simulink library "xpcnilib"  (Simulink 6.0)
settings: Solver=ode45  SolverMode=SingleTasking  StartTime=0.0  StopTime=10.0  RelTol=1e-3
undefined symbols (not defined in the file or in its folder): madnipcie, mctrnipcie, mctrnipciecap, mdacbisa, mdanipci670x, mdanipci671x, mdanipcie, mdionipci6527, mdionipcie, mencnipci660x, misa8255, mnigpib, mnipci660x, mpci8255
libraries: xpcmeasurementcomputinglib x6
(part 1 of 3)
settings Model: Creator=adowd  LastModifiedBy=gweast
settings DataIOCC: SignalLoggingName=logsOut
settings OptimizationCC: BooleanDataType=off
settings DebuggingCC: CheckExecutionContextPreStartOutputMsg=on  CheckExecutionContextRuntimeOutputMsg=on  SolverPrmCheckMsg=none
settings HardwareCC: TargetUnknown=on
settings SFSimCC: SFSimApplyToAllLibs=on  SFSimBuildMode=Incremental

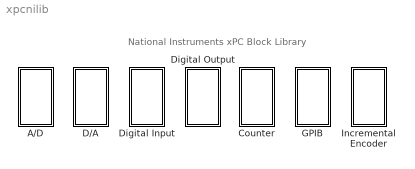
== system xpcnilib ==
  note: National Instruments xPC Block Library
  A/D : Subsystem  PropExecContextAcrossSSBoundary=on
  Counter : Subsystem  PropExecContextAcrossSSBoundary=on
  D/A : Subsystem  PropExecContextAcrossSSBoundary=on
  Digital Input : Subsystem  PropExecContextAcrossSSBoundary=on
  Digital Output : Subsystem  PropExecContextAcrossSSBoundary=on
  GPIB : Subsystem  PropExecContextAcrossSSBoundary=on
  Incremental Encoder : Subsystem  PropExecContextAcrossSSBoundary=on

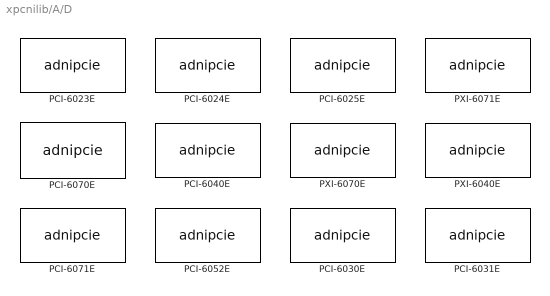
== system xpcnilib/A/D ==
  "PCI-6023E " : S-Function  InitFcn=madnipcie(1);  FunctionName=adnipcie  Parameters="channel, range, coupling, sampletime, slot,  boardType"  mask(adnipcie){channel=[1], range=[-10], coupling=[0], sampletime=0.001, slot=-1}
      mask prompts: channel "Channel vector:"; range "Range vector:"; coupling "Input coupling vector:"; sampletime "Sample time:"; slot "PCI slot (-1: autosearch):"
      mask help:
      | PCI-6023E
      | National Instruments
      | Analog Input
      mask init:
      | boardType=1;
      | madnipcie(2,channel, range, coupling, slot, boardType);
      mask Help: helpview(fullfile(docroot, 'mapfiles', 'xpc.map'), 'NationalInstruments_PCI-6023E_AD')
      mask Display: disp('PCI-6023E\nNational Instr.\nAnalog Input');port_label('output',1,'1');
  "PCI-6024E " : S-Function  InitFcn=madnipcie(1);  FunctionName=adnipcie  Parameters="channel, range, coupling, sampletime, slot,  boardType"  mask(adnipcie){channel=[1], range=[-10], coupling=[0], sampletime=0.001, slot=-1}
      mask prompts: channel "Channel vector:"; range "Range vector:"; coupling "Input coupling vector:"; sampletime "Sample time:"; slot "PCI slot (-1: autosearch):"
      mask help:
      | PCI-6024E
      | National Instruments
      | Analog Input
      mask init:
      | boardType=2;
      | madnipcie(2,channel, range, coupling, slot, boardType);
      mask Help: helpview(fullfile(docroot, 'mapfiles', 'xpc.map'), 'NationalInstruments_PCI-6024E_AD')
      mask Display: disp('PCI-6024E\nNational Instr.\nAnalog Input');port_label('output',1,'1');
  "PCI-6025E " : S-Function  InitFcn=madnipcie(1);  FunctionName=adnipcie  Parameters="channel, range, coupling, sampletime, slot,  boardType"  mask(adnipcie){channel=[1], range=[-10], coupling=[0], sampletime=0.001, slot=-1}
      mask prompts: channel "Channel vector:"; range "Range vector:"; coupling "Input coupling vector:"; sampletime "Sample time:"; slot "PCI slot (-1: autosearch):"
      mask help:
      | PCI-6025E
      | National Instruments
      | Analog Input
      mask init:
      | boardType=3;
      | madnipcie(2,channel, range, coupling, slot, boardType);
      mask Help: helpview(fullfile(docroot, 'mapfiles', 'xpc.map'), 'NationalInstruments_PCI-6025E_AD')
      mask Display: disp('PCI-6025E\nNational Instr.\nAnalog Input');port_label('output',1,'1');
  "PCI-6030E " : S-Function  InitFcn=madnipcie(1);  FunctionName=adnipcie  Parameters="channel, range, coupling, sampletime, slot,  boardType"  mask(adnipcie){channel=[1], range=[-10], coupling=[0], sampletime=0.001, slot=-1}
      mask prompts: channel "Channel vector:"; range "Range vector:"; coupling "Input coupling vector:"; sampletime "Sample time:"; slot "PCI slot (-1: autosearch):"
      mask help:
      | PCI-6030E
      | National Instruments
      | Analog Input
      mask init:
      | boardType=10;
      | madnipcie(2,channel, range, coupling, slot, boardType);
      mask Help: helpview(fullfile(docroot, 'mapfiles', 'xpc.map'), 'NationalInstruments_PCI-MIO-16XE-10_AD')
      mask Display: disp('PCI-6030E\nNational Instr.\nAnalog Input');port_label('output',1,'1');
  "PCI-6031E " : S-Function  InitFcn=madnipcie(1);  FunctionName=adnipcie  Parameters="channel, range, coupling, sampletime, slot,  boardType"  mask(adnipcie){channel=[1], range=[-10], coupling=[0], sampletime=0.001, slot=-1}
      mask prompts: channel "Channel vector:"; range "Range vector:"; coupling "Input coupling vector:"; sampletime "Sample time:"; slot "PCI slot (-1: autosearch):"
      mask help:
      | PCI-6031E
      | National Instruments
      | Analog Input
      mask init:
      | boardType=11;
      | madnipcie(2,channel, range, coupling, slot, boardType);
      mask Help: helpview(fullfile(docroot, 'mapfiles', 'xpc.map'), 'NationalInstruments_PCI-6031E_AD')
      mask Display: disp('PCI-6031E\nNational Instr.\nAnalog Input');port_label('output',1,'1');
  "PCI-6040E " : S-Function  InitFcn=madnipcie(1);  FunctionName=adnipcie  Parameters="channel, range, coupling, sampletime, slot,  boardType"  mask(adnipcie){channel=[1], range=[-10], coupling=[0], sampletime=0.001, slot=-1}
      mask prompts: channel "Channel vector:"; range "Range vector:"; coupling "Input coupling vector:"; sampletime "Sample time:"; slot "PCI slot (-1: autosearch):"
      mask help:
      | PCI-6040E
      | National Instruments
      | Analog Input
      mask init:
      | boardType=5;
      | madnipcie(2,channel, range, coupling, slot, boardType);
      mask Help: helpview(fullfile(docroot, 'mapfiles', 'xpc.map'), 'NationalInstruments_PCI-MIO-16E-4_AD')
      mask Display: disp('PCI-6040E\nNational Instr.\nAnalog Input');port_label('output',1,'1');
  "PCI-6052E " : S-Function  InitFcn=madnipcie(1);  FunctionName=adnipcie  Parameters="channel, range, coupling, sampletime, slot,  boardType"  mask(adnipcie){channel=[1], range=[-10], coupling=[0], sampletime=0.001, slot=-1}
      mask prompts: channel "Channel vector:"; range "Range vector:"; coupling "Input coupling vector:"; sampletime "Sample time:"; slot "PCI slot (-1: autosearch):"
      mask help:
      | PCI-6052E
      | National Instruments
      | Analog Input
      mask init:
      | boardType=9;
      | madnipcie(2,channel, range, coupling, slot, boardType);
      mask Help: helpview(fullfile(docroot, 'mapfiles', 'xpc.map'), 'NationalInstruments_PCI-6052E_AD')
      mask Display: disp('PCI-6052E\nNational Instr.\nAnalog Input');port_label('output',1,'1');
  "PCI-6070E " : S-Function  InitFcn=madnipcie(1);  FunctionName=adnipcie  Parameters="channel, range, coupling, sampletime, slot,  boardType"  mask(adnipcie){channel=[1], range=[-10], coupling=[0], sampletime=0.001, slot=-1}
      mask prompts: channel "Channel vector:"; range "Range vector:"; coupling "Input coupling vector:"; sampletime "Sample time:"; slot "PCI slot (-1: autosearch):"
      mask help:
      | PCI-6070E
      | National Instruments
      | Analog Input
      mask init:
      | boardType=4;
      | madnipcie(2,channel, range, coupling, slot, boardType);
      mask Help: helpview(fullfile(docroot, 'mapfiles', 'xpc.map'), 'NationalInstruments_PCI-MIO-16E-1_AD')
      mask Display: disp('PCI-6070E\nNational Instr.\nAnalog Input');port_label('output',1,'1');
  "PCI-6071E " : S-Function  InitFcn=madnipcie(1);  FunctionName=adnipcie  Parameters="channel, range, coupling, sampletime, slot,  boardType"  mask(adnipcie){channel=[1], range=[-10], coupling=[0], sampletime=0.001, slot=-1}
      mask prompts: channel "Channel vector:"; range "Range vector:"; coupling "Input coupling vector:"; sampletime "Sample time:"; slot "PCI slot (-1: autosearch):"
      mask help:
      | PCI-6071E
      | National Instruments
      | Analog Input
      mask init:
      | boardType=8;
      | madnipcie(2,channel, range, coupling, slot, boardType);
      mask Help: helpview(fullfile(docroot, 'mapfiles', 'xpc.map'), 'NationalInstruments_PCI-6071E_AD')
      mask Display: disp('PCI-6071E\nNational Instr.\nAnalog Input');port_label('output',1,'1');
  "PXI-6040E " : S-Function  InitFcn=madnipcie(1);  FunctionName=adnipcie  Parameters="channel, range, coupling, sampletime, slot,  boardType"  mask(adnipcie){channel=[1], range=[-10], coupling=[0], sampletime=0.001, slot=-1}
      mask prompts: channel "Channel vector:"; range "Range vector:"; coupling "Input coupling vector:"; sampletime "Sample time:"; slot "PCI slot (-1: autosearch):"
      mask help:
      | PXI-6040E
      | National Instruments
      | Analog Input
      mask init:
      | boardType=7;
      | madnipcie(2,channel, range, coupling, slot, boardType);
      mask Help: helpview(fullfile(docroot, 'mapfiles', 'xpc.map'), 'NationalInstruments_PXI-6040E_AD')
      mask Display: disp('PXI-6040E\nNational Instr.\nAnalog Input');port_label('output',1,'1');
  "PXI-6070E " : S-Function  InitFcn=madnipcie(1);  FunctionName=adnipcie  Parameters="channel, range, coupling, sampletime, slot,  boardType"  mask(adnipcie){channel=[1], range=[-10], coupling=[0], sampletime=0.001, slot=-1}
      mask prompts: channel "Channel vector:"; range "Range vector:"; coupling "Input coupling vector:"; sampletime "Sample time:"; slot "PCI slot (-1: autosearch):"
      mask help:
      | PXI-6070E
      | National Instruments
      | Analog Input
      mask init:
      | boardType=6;
      | madnipcie(2,channel, range, coupling, slot, boardType);
      mask Help: helpview(fullfile(docroot, 'mapfiles', 'xpc.map'), 'NationalInstruments_PXI-6070E_AD')
      mask Display: disp('PXI-6070E\nNational Instr.\nAnalog Input');port_label('output',1,'1');
  "PXI-6071E " : S-Function  InitFcn=madnipcie(1);  FunctionName=adnipcie  Parameters="channel, range, coupling, sampletime, slot,  boardType"  mask(adnipcie){channel=[1], range=[-10], coupling=[0], sampletime=0.001, slot=-1}
      mask prompts: channel "Channel vector:"; range "Range vector:"; coupling "Input coupling vector:"; sampletime "Sample time:"; slot "PCI slot (-1: autosearch):"
      mask help:
      | PXI-6071E
      | National Instruments
      | Analog Input
      mask init:
      | boardType=12;
      | madnipcie(2,channel, range, coupling, slot, boardType);
      mask Help: helpview(fullfile(docroot, 'mapfiles', 'xpc.map'), 'NationalInstruments_PXI-6071E_AD')
      mask Display: disp('PXI-6071E\nNational Instr.\nAnalog Input');port_label('output',1,'1');

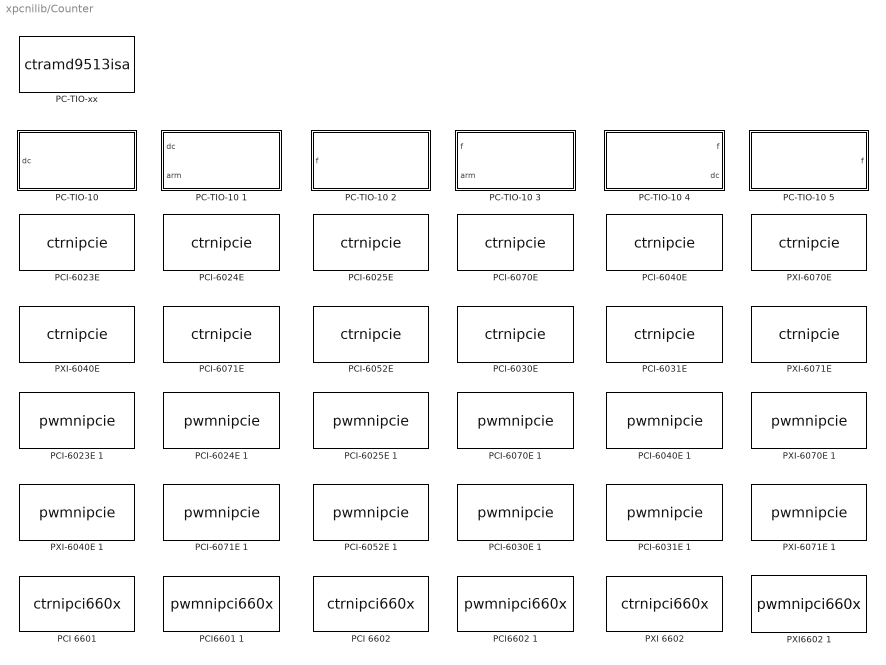
== system xpcnilib/Counter ==
  "PC-TIO-10 " : Subsystem  PropExecContextAcrossSSBoundary=on  mask(PWM){counterin=1, freq_base=F1=1MHz, freq=0.001, seq=High - Low, level=High, Ts=0.001, baseAddress=0x300}
      mask prompts: counterin "Counter:"; freq_base "Frequency base:"; freq "Relative output frequency:"; seq "Level sequence of square wave:"; level "Level when disarmed:"; Ts "Sample time:"; baseAddress "Base address (i.e. 0xd000):"
      mask help:
      | PC-TIO-10
      | National Instruments
      | PWM
      mask init:
      | init_arm=0;
      | initduty=0.5;
      | counter=counterin;
      | if counter>5
      | counter=counter-5;
      | baseAddress=['0x',dec2hex(hex2dec(baseAddress(3:end))+2)];
      | end;
      | [MasterMode, CounterMode, Init, Runtime, Term] =pwmarm_amd9513(counter, freq_base, freq, initduty, level, init_arm);
      | level=level-1;
      | seq=seq-1;
      mask Help: helpview(fullfile(docroot, 'mapfiles', 'xpc.map'), 'NationalInstruments_PC-TIO-10_Counter')
      mask StyleString: popup(1|2|3|4|5|6|7|8|9|10),popup(F1=1MHz|F2=100KHz|F3=10kHz|F4=1kHz|F5=100Hz),edit,popup(High - Low|Low- High),popup(Low|High),edit,edit
      mask Display: text(0.95,0.75,'PC-TIO-10','horizontalAlignment','right');text(0.95,0.50,'National Instr.','horizontalAlignment','right');text(0.95,0.25,'PWM','horizontalAlignment','right');port_label('input',1,[num2str(counterin),' (dc)'] );
  PC-TIO-10 1 : Subsystem  PropExecContextAcrossSSBoundary=on  mask(PWM){counterin=1, freq_base=F1=1MHz, freq=0.001, seq=High - Low, level=High, Ts=0.001, baseAddress=0x300}
      mask prompts: counterin "Counter:"; freq_base "Frequency base:"; freq "Relative output frequency:"; seq "Level sequence of square wave:"; level "Level when disarmed:"; Ts "Sample time:"; baseAddress "Base address (i.e. 0xd000):"
      mask help:
      | PC-TIO-10
      | National Instruments
      | PWM & ARM
      mask init: same as xpcnilib/Counter/PC-TIO-10 
      mask Help: helpview(fullfile(docroot, 'mapfiles', 'xpc.map'), 'NationalInstruments_PC-TIO-10-1_Counter')
      mask StyleString: popup(1|2|3|4|5|6|7|8|9|10),popup(F1=1MHz|F2=100KHz|F3=10kHz|F4=1kHz|F5=100Hz),edit,popup(High - Low|Low- High),popup(Low|High),edit,edit
      mask Display: text(0.95,0.75,'PC-TIO-10','horizontalAlignment','right');text(0.95,0.50,'National Instr.','horizontalAlignment','right');text(0.95,0.25,'PWM & ARM','horizontalAlignment','right');port_label('input',1,[num2str(counterin),' (dc)'] );port_label('input',2,[num2str(counterin),' (arm)'] );
  PC-TIO-10 2 : Subsystem  PropExecContextAcrossSSBoundary=on  mask(PWM){counterin=1, freq_base=F1=1MHz, duty=0.001, seq=High - Low, level=High, Ts=0.001, baseAddress=0x300}
      mask prompts: counterin "Counter:"; freq_base "Frequency base:"; duty "Output duty cycle:"; seq "Level sequence of square wave:"; level "Level when disarmed:"; Ts "Sample time:"; baseAddress "Base address (i.e. 0xd000):"
      mask help:
      | PC-TIO-10
      | National Instruments
      | FM
      mask init:
      | init_arm=0;
      | initfreq=0.005;
      | counter=counterin;
      | if counter>5
      | counter=counter-5;
      | baseAddress=['0x',dec2hex(hex2dec(baseAddress(3:end))+2)];
      | end;
      | [MasterMode, CounterMode, Init, Runtime, Term] =fmarm_amd9513(counter, freq_base, duty, initfreq, level, init_arm);
      | level=level-1;
      | seq=seq-1;
      mask Help: helpview(fullfile(docroot, 'mapfiles', 'xpc.map'), 'NationalInstruments_PC-TIO-10-2_Counter')
      mask StyleString: popup(1|2|3|4|5|6|7|8|9|10),popup(F1=1MHz|F2=100KHz|F3=10kHz|F4=1kHz|F5=100Hz),edit,popup(High - Low|Low- High),popup(Low|High),edit,edit
      mask Display: text(0.95,0.75,'PC-TIO-10','horizontalAlignment','right');text(0.95,0.50,'National Instr.','horizontalAlignment','right');text(0.95,0.25,'FM','horizontalAlignment','right');port_label('input',1,[num2str(counterin),' (f)'] );
  PC-TIO-10 3 : Subsystem  PropExecContextAcrossSSBoundary=on  mask(FM){counterin=1, freq_base=F1=1MHz, duty=0.001, seq=High - Low, level=High, Ts=0.001, baseAddress=0x300}
      mask prompts: counterin "Counter:"; freq_base "Frequency base:"; duty "Output duty cycle:"; seq "Level sequence of square wave:"; level "Level when disarmed:"; Ts "Sample time:"; baseAddress "Base address (i.e. 0xd000):"
      mask help:
      | PC-TIO-10
      | National Instruments
      | FM & ARM
      mask init: same as xpcnilib/Counter/PC-TIO-10 2
      mask Help: helpview(fullfile(docroot, 'mapfiles', 'xpc.map'), 'NationalInstruments_PC-TIO-10-3_Counter')
      mask StyleString: popup(1|2|3|4|5|6|7|8|9|10),popup(F1=1MHz|F2=100KHz|F3=10kHz|F4=1kHz|F5=100Hz),edit,popup(High - Low|Low- High),popup(Low|High),edit,edit
      mask Display: text(0.95,0.75,'PC-TIO-10','horizontalAlignment','right');text(0.95,0.50,'National Instr.','horizontalAlignment','right');text(0.95,0.25,'FM & ARM','horizontalAlignment','right');port_label('input',1,[num2str(counterin),' (f)'] );port_label('input',2,[num2str(counterin),' (arm)'] );
  PC-TIO-10 4 : Subsystem  PropExecContextAcrossSSBoundary=on  mask(PWMcap){counterin=1&2, freq_base=F1=1MHz, Ts=0.001, baseAddress=0x300}
      mask prompts: counterin "Counter:"; freq_base "Frequency base:"; Ts "Sample time:"; baseAddress "Base address (i.e. 0xd000):"
      mask help:
      | PC-TIO-10
      | National Instruments
      | PWM capture
      mask init:
      | counter=counterin;
      | if counter>4
      | counter=counter-4;
      | baseAddress=['0x',dec2hex(hex2dec(baseAddress(3:end))+2)];
      | end;
      | [MasterMode, CounterMode, Init, Runtime, Term] =pwmcap_amd9513(counter, freq_base);
      mask Help: helpview(fullfile(docroot, 'mapfiles', 'xpc.map'), 'NationalInstruments_PC-TIO-10-4_Counter')
      mask StyleString: popup(1&2|2&3|3&4|4&5|6&7|7&8|8&9|9&10),popup(F1=1MHz|F2=100KHz|F3=10kHz|F4=1kHz|F5=100Hz),edit,edit
      mask Display: text(0.05,0.75,'PC-TIO-10','horizontalAlignment','left');text(0.05,0.50,'National Instr.','horizontalAlignment','left');text(0.05,0.25,'PWM capture','horizontalAlignment','left');port_label('output',1,[num2str(counterin),' (f)'] );port_label('output',2,[num2str(counterin+1),' (dc)'] );
  PC-TIO-10 5 : Subsystem  PropExecContextAcrossSSBoundary=on  mask(FREQcap){counterin=1, freq_base=F1=1MHz, Ts=0.001, baseAddress=0x300}
      mask prompts: counterin "Counter:"; freq_base "Frequency base:"; Ts "Sample time:"; baseAddress "Base address (i.e. 0xd000):"
      mask help:
      | PC-TIO-10
      | National Instruments
      | Frequency capture
      mask init:
      | counter=counterin;
      | if counter>5
      | counter=counter-5;
      | baseAddress=['0x',dec2hex(hex2dec(baseAddress(3:end))+2)];
      | end;
      | [MasterMode, CounterMode, Init, Runtime, Term] =freqcap_amd9513(counter, freq_base);
      mask Help: helpview(fullfile(docroot, 'mapfiles', 'xpc.map'), 'NationalInstruments_PC-TIO-10-5_Counter')
      mask StyleString: popup(1|2|3|4|5|6|7|8|9|10),popup(F1=1MHz|F2=100KHz|F3=10kHz|F4=1kHz|F5=100Hz),edit,edit
      mask Display: text(0.05,0.75,'PC-TIO-10','horizontalAlignment','left');text(0.05,0.50,'National Instr.','horizontalAlignment','left');text(0.05,0.25,'Freq. capture','horizontalAlignment','left');port_label('output',1,[num2str(counterin),' (f)'] );
  "PC-TIO-xx " : S-Function  FunctionName=ctramd9513isa  Parameters=io, mm, cms, initir, ir, termir, ts, baseAddress  mask(pctioxx){mastermode=[], countermode=[], init=[], commands=[], term=[], ts=0.001, baseAddress='0x300'}
      mask prompts: mastermode "Master mode structure:"; countermode "Counter mode structure:"; init "Initialization command structure:"; commands "Runtime command structure:"; term "Termination command structure:"; ts "Sample time:"; baseAddress "9513 chip base address (i.e. 0xd000):"
      mask help:
      | PC-TIO-xx
      | National Instruments
      | AMD9513 Counter
      mask init:
      | baseAddress=hex2dec(baseAddress(3:end));
      | [io,mm, cms, initir, ir, termir]=mamd9513parse(mastermode, countermode, init, commands, term);
      mask Help: helpview(fullfile(docroot, 'mapfiles', 'xpc.map'), 'NationalInstruments_PC-TIO-xx_Counter')
      mask Display: disp('AMD9513\nCounter')
  "PCI 6601 " : S-Function  InitFcn=mnipci660x(1);  FunctionName=ctrnipci660x  Parameters=channel, sampletime, slot, initHigh, initLow, boardType  mask(ctrnipci6601){channel=1, initHigh=4000, initLow=4000, sampletime=-1, slot=-1}
      mask prompts: initHigh "Initial high count:"; initLow "Initial low count"; sampletime "Sample time:"; slot "PCI slot (-1: autosearch):"
      mask help:
      | PCI-6601
      | National Instruments
      | Pulse Generation
      mask init:
      | channel = channel - 1;
      | boardType = 3;
      | mnipci660x(2, channel, slot, boardType);
      mask Help: helpview(fullfile(docroot, 'mapfiles', 'xpc.map'), 'NationalInstruments_PCI-6601_CTR')
      mask StyleString: popup(1|2|3|4),edit,edit,edit,edit
      mask Display:
      | disp('PCI-6601\nNational Instr.\nPulse Gen.');
      | port_label('input', 1, 'H');
      | port_label('input', 2, 'L');
  "PCI 6602 " : S-Function  InitFcn=mnipci660x(1);  FunctionName=ctrnipci660x  Parameters=channel, sampletime, slot, initHigh, initLow, boardType  mask(ctrnipci6602){channel=1, initHigh=4000, initLow=4000, sampletime=-1, slot=-1}
      mask prompts: initHigh "Initial high count:"; initLow "Initial low count:"; sampletime "Sample time:"; slot "PCI slot (-1: autosearch):"
      mask help:
      | PCI-6602
      | National Instruments
      | Pulse Generation
      mask init:
      | channel = channel - 1;
      | boardType = 1;
      | mnipci660x(2, channel, slot, boardType);
      mask Help: helpview(fullfile(docroot, 'mapfiles', 'xpc.map'), 'NationalInstruments_PCI-6602_CTR')
      mask StyleString: popup(1|2|3|4|5|6|7|8),edit,edit,edit,edit
      mask Display:
      | disp('PCI-6602\nNational Instr.\nPulse Gen');
      | port_label('input', 1, 'H');
      | port_label('input', 2, 'L');
  "PCI-6023E " : S-Function  InitFcn=mctrnipcie(1);  FunctionName=ctrnipcie  Parameters=channel, sampletime, slot, boardType  mask(ctrnipci6023e){channel=Counter 0, sampletime=-1, slot=-1}
      mask prompts: channel "Counter:"; sampletime "Sample time:"; slot "PCI slot (-1: autosearch):"
      mask help:
      | PCI-6023E
      | National Instruments
      | Pulse Generation
      mask init:
      | boardType = 1;
      | mctrnipcie(2, boardType, slot, channel);
      mask Help: helpview(fullfile(docroot, 'mapfiles', 'xpc.map'),'NationalInstruments_PCI-6023E_CTR');
      mask StyleString: popup(Counter 0|Counter 1|Both),edit,edit
      mask Display: disp('PCI-6023E\nNational Instr.\nPulse Gen.');port_label('input', 1, '0');
  PCI-6023E 1 : S-Function  InitFcn=mctrnipciecap(1);  FunctionName=pwmnipcie  Parameters=channel, trigmd, polarity, tsamp, slot, boardType  mask(pwmnipci6023e){channel=0, trigmd=Level Triggered, polarity=Active low, tsamp=0.01, slot=-1}
      mask prompts: channel "Counter:"; trigmd "Trigger mode:"; tsamp "Sample time:"; slot "PCI slot (-1: autosearch):"
      mask help:
      | PCI-6023E
      | National Instruments
      | Pulsewidth/Period measurement
      mask init:
      | boardType = 1;
      | 
      | channel  = channel  - 1;
      | trigmd   = trigmd   - 1;
      | polarity = polarity - 1;
      | mctrnipciecap(2, boardType, slot, channel);
      mask Help: helpview(fullfile(docroot, 'mapfiles', 'xpc.map'),'NationalInstruments_PCI-6023E_CTRMEAS');
      mask StyleString: popup(0|1),popup(Level Triggered|Edge Triggered),popup(Active low|Active high),edit,edit
      mask CallbackString: |mnipwmmaskenable(gcb)|||
      mask Display: disp('PCI-6023E\nNational Instr.\nPulsewidth/Period Meas.');port_label('output', 1, '0');
  "PCI-6024E " : S-Function  FunctionName=ctrnipcie  Parameters=channel, sampletime, slot, boardType  mask(ctrnipci6024e){channel=Counter 0, sampletime=-1, slot=-1}
      mask prompts: channel "Counter:"; sampletime "Sample time:"; slot "PCI slot (-1: autosearch):"
      mask help:
      | PCI-6024E
      | National Instruments
      | Pulse Generation
      mask init:
      | boardType = 2;
      | mctrnipcie(2, boardType, slot, channel);
      mask Help: helpview(fullfile(docroot, 'mapfiles', 'xpc.map'),'NationalInstruments_PCI-6024E_CTR');
      mask StyleString: popup(Counter 0|Counter 1|Both),edit,edit
      mask Display: disp('PCI-6024E\nNational Instr.\nPulse Gen.');port_label('input', 1, '0');
  PCI-6024E 1 : S-Function  InitFcn=mctrnipciecap(1);  FunctionName=pwmnipcie  Parameters=channel, trigmd, polarity, tsamp, slot, boardType  mask(pwmnipci6024e){channel=0, trigmd=Level Triggered, polarity=Active low, tsamp=0.01, slot=-1}
      mask prompts: channel "Counter:"; trigmd "Trigger mode:"; tsamp "Sample time:"; slot "PCI slot (-1: autosearch):"
      mask help:
      | PCI-6024E
      | National Instruments
      | Pulsewidth/Period measurement
      mask init:
      | boardType = 2;
      | 
      | channel  = channel  - 1;
      | trigmd   = trigmd   - 1;
      | polarity = polarity - 1;
      | mctrnipciecap(2, boardType, slot, channel);
      mask Help: helpview(fullfile(docroot, 'mapfiles', 'xpc.map'),'NationalInstruments_PCI-6024E_CTRMEAS');
      mask StyleString: popup(0|1),popup(Level Triggered|Edge Triggered),popup(Active low|Active high),edit,edit
      mask CallbackString: |mnipwmmaskenable(gcb)|||
      mask Display: disp('PCI-6024E\nNational Instr.\nPulsewidth/Period Meas.');port_label('output', 1, '0');
  "PCI-6025E " : S-Function  FunctionName=ctrnipcie  Parameters=channel, sampletime, slot, boardType  mask(ctrnipci6025e){channel=Counter 0, sampletime=-1, slot=-1}
      mask prompts: channel "Counter:"; sampletime "Sample time:"; slot "PCI slot (-1: autosearch):"
      mask help:
      | PCI-6025E
      | National Instruments
      | Pulse Generation
      mask init:
      | boardType = 3;
      | mctrnipcie(2, boardType, slot, channel);
      mask Help: helpview(fullfile(docroot, 'mapfiles', 'xpc.map'),'NationalInstruments_PCI-6025E_CTR');
      mask StyleString: popup(Counter 0|Counter 1|Both),edit,edit
      mask Display: disp('PCI-6025E\nNational Instr.\nPulse Gen.');port_label('input', 1, '0');
  PCI-6025E 1 : S-Function  InitFcn=mctrnipciecap(1);  FunctionName=pwmnipcie  Parameters=channel, trigmd, polarity, tsamp, slot, boardType  mask(pwmnipci6025e){channel=0, trigmd=Level Triggered, polarity=Active low, tsamp=0.01, slot=-1}
      mask prompts: channel "Counter:"; trigmd "Trigger mode:"; tsamp "Sample time:"; slot "PCI slot (-1: autosearch):"
      mask help:
      | PCI-6025E
      | National Instruments
      | Pulsewidth/Period measurement
      mask init:
      | boardType = 3;
      | 
      | channel  = channel  - 1;
      | trigmd   = trigmd   - 1;
      | polarity = polarity - 1;
      | mctrnipciecap(2, boardType, slot, channel);
      mask Help: helpview(fullfile(docroot, 'mapfiles', 'xpc.map'),'NationalInstruments_PCI-6025E_CTRMEAS');
      mask StyleString: popup(0|1),popup(Level Triggered|Edge Triggered),popup(Active low|Active high),edit,edit
      mask CallbackString: |mnipwmmaskenable(gcb)|||
      mask Display: disp('PCI-6025E\nNational Instr.\nPulsewidth/Period Meas.');port_label('output', 1, '0');
  "PCI-6030E " : S-Function  FunctionName=ctrnipcie  Parameters=channel, sampletime, slot, boardType  mask(ctrnipci6030e){channel=Counter 0, sampletime=-1, slot=-1}
      mask prompts: channel "Counter:"; sampletime "Sample time:"; slot "PCI slot (-1: autosearch):"
      mask help:
      | PCI-6030E
      | National Instruments
      | Pulse Generation
      mask init:
      | boardType = 10;
      | mctrnipcie(2, boardType, slot, channel);
      mask Help: helpview(fullfile(docroot, 'mapfiles', 'xpc.map'),'NationalInstruments_PCI-MIO-16XE-10_CTR');
      mask StyleString: popup(Counter 0|Counter 1|Both),edit,edit
      mask Display: disp('PCI-6030E\nNational Instr.\nPulse Gen.');port_label('input', 1, '0');
  PCI-6030E 1 : S-Function  InitFcn=mctrnipciecap(1);  FunctionName=pwmnipcie  Parameters=channel, trigmd, polarity, tsamp, slot, boardType  mask(pwmnipci6030e){channel=0, trigmd=Level Triggered, polarity=Active low, tsamp=0.01, slot=-1}
      mask prompts: channel "Counter:"; trigmd "Trigger mode:"; tsamp "Sample time:"; slot "PCI slot (-1: autosearch):"
      mask help:
      | PCI-6030E
      | National Instruments
      | Pulsewidth/Period measurement
      mask init:
      | boardType = 10;
      | 
      | channel  = channel  - 1;
      | trigmd   = trigmd   - 1;
      | polarity = polarity - 1;
      | mctrnipciecap(2, boardType, slot, channel);
      mask Help: helpview(fullfile(docroot, 'mapfiles', 'xpc.map'),'NationalInstruments_PCI-MIO-16XE-10_CTRMEAS');
      mask StyleString: popup(0|1),popup(Level Triggered|Edge Triggered),popup(Active low|Active high),edit,edit
      mask CallbackString: |mnipwmmaskenable(gcb)|||
      mask Display: disp('PCI-6030E\nNational Instr.\nPulsewidth/Period Meas.');port_label('output', 1, '0');
  "PCI-6031E " : S-Function  FunctionName=ctrnipcie  Parameters=channel, sampletime, slot, boardType  mask(ctrnipci6031e){channel=Counter 0, sampletime=-1, slot=-1}
      mask prompts: channel "Counter:"; sampletime "Sample time:"; slot "PCI slot (-1: autosearch):"
      mask help:
      | PCI-6031E
      | National Instruments
      | Pulse Generation
      mask init:
      | boardType = 11;
      | mctrnipcie(2, boardType, slot, channel);
      mask Help: helpview(fullfile(docroot, 'mapfiles', 'xpc.map'),'NationalInstruments_PCI-6031E_CTR');
      mask StyleString: popup(Counter 0|Counter 1|Both),edit,edit
      mask Display: disp('PCI-6031E\nNational Instr.\nPulse Gen.');port_label('input', 1, '0');
  PCI-6031E 1 : S-Function  InitFcn=mctrnipciecap(1);  FunctionName=pwmnipcie  Parameters=channel, trigmd, polarity, tsamp, slot, boardType  mask(pwmnipci6031e){channel=0, trigmd=Level Triggered, polarity=Active low, tsamp=0.01, slot=-1}
      mask prompts: channel "Counter:"; trigmd "Trigger mode:"; tsamp "Sample time:"; slot "PCI slot (-1: autosearch):"
      mask help:
      | PCI-6031E
      | National Instruments
      | Pulsewidth/Period measurement
      mask init:
      | boardType = 11;
      | 
      | channel  = channel  - 1;
      | trigmd   = trigmd   - 1;
      | polarity = polarity - 1;
      | mctrnipciecap(2, boardType, slot, channel);
      mask Help: helpview(fullfile(docroot, 'mapfiles', 'xpc.map'),'NationalInstruments_PCI-6031E_CTRMEAS');
      mask StyleString: popup(0|1),popup(Level Triggered|Edge Triggered),popup(Active low|Active high),edit,edit
      mask CallbackString: |mnipwmmaskenable(gcb)|||
      mask Display: disp('PCI-6031E\nNational Instr.\nPulsewidth/Period Meas.');port_label('output', 1, '0');
  PCI-6040E : S-Function  FunctionName=ctrnipcie  Parameters=channel, sampletime, slot, boardType  mask(ctrnipci6040e){channel=Counter 0, sampletime=-1, slot=-1}
      mask prompts: channel "Counter:"; sampletime "Sample time:"; slot "PCI slot (-1: autosearch):"
      mask help:
      | PCI-6040E
      | National Instruments
      | Pulse Generation
      mask init:
      | boardType = 5;
      | mctrnipcie(2, boardType, slot, channel);
      mask Help: helpview(fullfile(docroot, 'mapfiles', 'xpc.map'),'NationalInstruments_PCI-MIO-16E-4_CTR');
      mask StyleString: popup(Counter 0|Counter 1|Both),edit,edit
      mask Display: disp('PCI-6040E\nNational Instr.\nPulse Gen.');port_label('input', 1, '0');
  PCI-6040E 1 : S-Function  InitFcn=mctrnipciecap(1);  FunctionName=pwmnipcie  Parameters=channel, trigmd, polarity, tsamp, slot, boardType  mask(pwmnipci6040e){channel=0, trigmd=Level Triggered, polarity=Active low, tsamp=0.01, slot=-1}
      mask prompts: channel "Counter:"; trigmd "Trigger mode:"; tsamp "Sample time:"; slot "PCI slot (-1: autosearch):"
      mask help:
      | PCI-6040E
      | National Instruments
      | Pulsewidth/Period measurement
      mask init:
      | boardType = 5;
      | 
      | channel  = channel  - 1;
      | trigmd   = trigmd   - 1;
      | polarity = polarity - 1;
      | mctrnipciecap(2, boardType, slot, channel);
      mask Help: helpview(fullfile(docroot, 'mapfiles', 'xpc.map'),'NationalInstruments_PCI-MIO-16E-4_CTRMEAS');
      mask StyleString: popup(0|1),popup(Level Triggered|Edge Triggered),popup(Active low|Active high),edit,edit
      mask CallbackString: |mnipwmmaskenable(gcb)|||
      mask Display: disp('PCI-6040E\nNational Instr.\nPulsewidth/Period Meas.');port_label('output', 1, '0');
  "PCI-6052E " : S-Function  FunctionName=ctrnipcie  Parameters=channel, sampletime, slot, boardType  mask(ctrnipci6052e){channel=Counter 0, sampletime=-1, slot=-1}
      mask prompts: channel "Counter:"; sampletime "Sample time:"; slot "PCI slot (-1: autosearch):"
      mask help:
      | PCI-6052E
      | National Instruments
      | Pulse Generation
      mask init:
      | boardType = 9;
      | mctrnipcie(2, boardType, slot, channel);
      mask Help: helpview(fullfile(docroot, 'mapfiles', 'xpc.map'),'NationalInstruments_PCI-6052E_CTR');
      mask StyleString: popup(Counter 0|Counter 1|Both),edit,edit
      mask Display: disp('PCI-6052E\nNational Instr.\nPulse Gen.');port_label('input', 1, '0');
  PCI-6052E 1 : S-Function  InitFcn=mctrnipciecap(1);  FunctionName=pwmnipcie  Parameters=channel, trigmd, polarity, tsamp, slot, boardType  mask(pwmnipci6025e){channel=0, trigmd=Level Triggered, polarity=Active low, tsamp=0.01, slot=-1}
      mask prompts: channel "Counter:"; trigmd "Trigger mode:"; tsamp "Sample time:"; slot "PCI slot (-1: autosearch):"
      mask help:
      | PCI-6052E
      | National Instruments
      | Pulsewidth/Period measurement
      mask init:
      | boardType = 9;
      | 
      | channel  = channel  - 1;
      | trigmd   = trigmd   - 1;
      | polarity = polarity - 1;
      | mctrnipciecap(2, boardType, slot, channel);
      mask Help: helpview(fullfile(docroot, 'mapfiles', 'xpc.map'),'NationalInstruments_PCI-6052E_CTRMEAS');
      mask StyleString: popup(0|1),popup(Level Triggered|Edge Triggered),popup(Active low|Active high),edit,edit
      mask CallbackString: |mnipwmmaskenable(gcb)|||
      mask Display: disp('PCI-6052E\nNational Instr.\nPulsewidth/Period Meas.');port_label('output', 1, '0');
  "PCI-6070E " : S-Function  FunctionName=ctrnipcie  Parameters=channel, sampletime, slot, boardType  mask(ctrnipci6070e){channel=Counter 0, sampletime=-1, slot=-1}
      mask prompts: channel "Counter:"; sampletime "Sample time:"; slot "PCI slot (-1: autosearch):"
      mask help:
      | PCI-6070E
      | National Instruments
      | Pulse Generation
      mask init:
      | boardType = 4;
      | mctrnipcie(2, boardType, slot, channel);
      mask Help: helpview(fullfile(docroot, 'mapfiles', 'xpc.map'),'NationalInstruments_PCI-MIO-16E-1_CTR');
      mask StyleString: popup(Counter 0|Counter 1|Both),edit,edit
      mask Display: disp('PCI-6070E\nNational Instr.\nPulse Gen.');port_label('input', 1, '0');
  PCI-6070E 1 : S-Function  InitFcn=mctrnipciecap(1);  FunctionName=pwmnipcie  Parameters=channel, trigmd, polarity, tsamp, slot, boardType  mask(pwmnipci6070e){channel=0, trigmd=Level Triggered, polarity=Active low, tsamp=0.01, slot=-1}
      mask prompts: channel "Counter:"; trigmd "Trigger mode:"; tsamp "Sample time:"; slot "PCI slot (-1: autosearch):"
      mask help:
      | PCI-6070E
      | National Instruments
      | Pulsewidth/Period measurement
      mask init:
      | boardType = 4;
      | 
      | channel  = channel  - 1;
      | trigmd   = trigmd   - 1;
      | polarity = polarity - 1;
      | mctrnipciecap(2, boardType, slot, channel);
      mask Help: helpview(fullfile(docroot, 'mapfiles', 'xpc.map'),'NationalInstruments_PCI-MIO-16E-1_CTRMEAS');
      mask StyleString: popup(0|1),popup(Level Triggered|Edge Triggered),popup(Active low|Active high),edit,edit
      mask CallbackString: |mnipwmmaskenable(gcb)|||
      mask Display: disp('PCI-6070E\nNational Instr.\nPulsewidth/Period Meas.');port_label('output', 1, '0');
  "PCI-6071E " : S-Function  FunctionName=ctrnipcie  Parameters=channel, sampletime, slot, boardType  mask(ctrnipci6071e){channel=Counter 0, sampletime=-1, slot=-1}
      mask prompts: channel "Counter:"; sampletime "Sample time:"; slot "PCI slot (-1: autosearch):"
      mask help:
      | PCI-6071E
      | National Instruments
      | Pulse Generation
      mask init:
      | boardType = 8;
      | mctrnipcie(2, boardType, slot, channel);
      mask Help: helpview(fullfile(docroot, 'mapfiles', 'xpc.map'),'NationalInstruments_PCI-6071E_CTR');
      mask StyleString: popup(Counter 0|Counter 1|Both),edit,edit
      mask Display: disp('PCI-6071E\nNational Instr.\nPulse Gen.');port_label('input', 1, '0');
  PCI-6071E 1 : S-Function  InitFcn=mctrnipciecap(1);  FunctionName=pwmnipcie  Parameters=channel, trigmd, polarity, tsamp, slot, boardType  mask(pwmnipci6071e){channel=0, trigmd=Level Triggered, polarity=Active low, tsamp=0.01, slot=-1}
      mask prompts: channel "Counter:"; trigmd "Trigger mode:"; tsamp "Sample time:"; slot "PCI slot (-1: autosearch):"
      mask help:
      | PCI-6071E
      | National Instruments
      | Pulsewidth/Period measurement
      mask init:
      | boardType = 8;
      | 
      | channel  = channel  - 1;
      | trigmd   = trigmd   - 1;
      | polarity = polarity - 1;
      | mctrnipciecap(2, boardType, slot, channel);
      mask Help: helpview(fullfile(docroot, 'mapfiles', 'xpc.map'),'NationalInstruments_PCI-6071E_CTRMEAS');
      mask StyleString: popup(0|1),popup(Level Triggered|Edge Triggered),popup(Active low|Active high),edit,edit
      mask CallbackString: |mnipwmmaskenable(gcb)|||
      mask Display: disp('PCI-6071E\nNational Instr.\nPulsewidth/Period Meas.');port_label('output', 1, '0');
  PCI6601 1 : S-Function  InitFcn=mnipci660x(1);  FunctionName=pwmnipci660x  Parameters=channel, trigmd, polarity, tsamp, slot, boardType  mask(pwmnipci6601){channel=1, trigmd=Level Triggered, polarity=Active Low, tsamp=0.001, slot=-1}
      mask prompts: trigmd "Trigger mode:"; tsamp "Sample time:"; slot "PCI slot (-1: autosearch):"
      mask help:
      | PCI-6601
      | National Instruments
      | Pulsewidth/Period Measurement
      mask init:
      | boardType = 3;
      | 
      | channel  = channel  - 1;
      | trigmd   = trigmd   - 1;
      | polarity = polarity - 1;
      | mnipci660x(2, channel, slot, boardType );
      mask Help: helpview(fullfile(docroot, 'mapfiles', 'xpc.map'), 'NationalInstruments_PCI-6601_CTRMEAS')
      mask StyleString: popup(1|2|3|4),popup(Level Triggered|Edge Triggered),popup(Active Low|Active High),edit,edit
      mask CallbackString: |mnipwmmaskenable(gcb);|||
      mask Display:
      | disp('PCI-6601\nNational Instr.\nPulsewidth/Period Meas.');
      | port_label('output', 1, 'C');
  PCI6602 1 : S-Function  InitFcn=mnipci660x(1);  FunctionName=pwmnipci660x  Parameters=channel, trigmd, polarity, tsamp, slot, boardType  mask(pwmnipci6602){channel=1, trigmd=Level Triggered, polarity=Active Low, tsamp=0.001, slot=-1}
      mask prompts: trigmd "Trigger mode:"; tsamp "Sample time:"; slot "PCI slot (-1: autosearch):"
      mask help:
      | PCI-6602
      | National Instruments
      | Pulsewidth/Period Measurement
      mask init:
      | boardType = 1;
      | 
      | channel  = channel  - 1;
      | trigmd   = trigmd   - 1;
      | polarity = polarity - 1;
      | mnipci660x( 2, channel, slot, boardType )
      mask Help: helpview(fullfile(docroot, 'mapfiles', 'xpc.map'), 'NationalInstruments_PCI-6602_CTRMEAS')
      mask StyleString: popup(1|2|3|4|5|6|7|8),popup(Level Triggered|Edge Triggered),popup(Active Low|Active High),edit,edit
      mask CallbackString: |mnipwmmaskenable(gcb);|||
      mask Display:
      | disp('PCI-6602\nNational Instr.\nPulsewidth/Period Meas.');
      | port_label('output', 1, 'C');
  "PXI 6602 " : S-Function  InitFcn=mnipci660x(1);  FunctionName=ctrnipci660x  Parameters=channel, sampletime, slot, initHigh, initLow, boardType  mask(ctrnipxi6602){channel=1, initHigh=4000, initLow=4000, sampletime=-1, slot=-1}
      mask prompts: initHigh "Initial high count:"; initLow "Initial low count:"; sampletime "Sample time:"; slot "PCI slot (-1: autosearch):"
      mask help:
      | PXI-6602
      | National Instruments
      | Pulse Generation
      mask init:
      | channel = channel - 1;
      | boardType = 2;
      | mnipci660x(2, channel, slot, boardType);
      mask Help: helpview(fullfile(docroot, 'mapfiles', 'xpc.map'), 'NationalInstruments_PCI-6602_CTR')
      mask StyleString: popup(1|2|3|4|5|6|7|8),edit,edit,edit,edit
      mask Display:
      | disp('PXI-6602\nNational Instr.\nPulse Gen.');
      | port_label('input', 1, 'H' );
      | port_label('input', 2, 'L' );
  "PXI-6040E " : S-Function  FunctionName=ctrnipcie  Parameters=channel, sampletime, slot, boardType  mask(ctrnipxi6040e){channel=Counter 0, sampletime=-1, slot=-1}
      mask prompts: channel "Counter:"; sampletime "Sample time:"; slot "PCI slot (-1: autosearch):"
      mask help:
      | PXI-6040E
      | National Instruments
      | Pulse Generation
      mask init:
      | boardType = 7;
      | mctrnipcie(2, boardType, slot, channel);
      mask Help: helpview(fullfile(docroot, 'mapfiles', 'xpc.map'),'NationalInstruments_PXI-6040E_CTR');
      mask StyleString: popup(Counter 0|Counter 1|Both),edit,edit
      mask Display: disp('PXI-6040E\nNational Instr.\nPulse Gen.');port_label('input', 1, '0');
  PXI-6040E 1 : S-Function  InitFcn=mctrnipciecap(1);  FunctionName=pwmnipcie  Parameters=channel, trigmd, polarity, tsamp, slot, boardType  mask(pwmnipxi6040e){channel=0, trigmd=Level Triggered, polarity=Active low, tsamp=0.01, slot=-1}
      mask prompts: channel "Counter:"; trigmd "Trigger mode:"; tsamp "Sample time:"; slot "PCI slot (-1: autosearch):"
      mask help:
      | PXI-6040E
      | National Instruments
      | Pulsewidth/Period measurement
      mask init:
      | boardType = 7;
      | 
      | channel  = channel  - 1;
      | trigmd   = trigmd   - 1;
      | polarity = polarity - 1;
      | mctrnipciecap(2, boardType, slot, channel);
      mask Help: helpview(fullfile(docroot, 'mapfiles', 'xpc.map'),'NationalInstruments_PXI-6040E_CTRMEAS');
      mask StyleString: popup(0|1),popup(Level Triggered|Edge Triggered),popup(Active low|Active high),edit,edit
      mask CallbackString: |mnipwmmaskenable(gcb)|||
      mask Display: disp('PXI-6040E\nNational Instr.\nPulsewidth/Period Meas.');port_label('output', 1, '0');
  "PXI-6070E " : S-Function  FunctionName=ctrnipcie  Parameters=channel, sampletime, slot, boardType  mask(ctrnipxi6070e){channel=Counter 0, sampletime=-1, slot=-1}
      mask prompts: channel "Counter:"; sampletime "Sample time:"; slot "PCI slot (-1: autosearch):"
      mask help:
      | PXI-6070E
      | National Instruments
      | Pulse Generation
      mask init:
      | boardType = 6;
      | mctrnipcie(2, boardType, slot, channel);
      mask Help: helpview(fullfile(docroot, 'mapfiles', 'xpc.map'),'NationalInstruments_PXI-6070E_CTR');
      mask StyleString: popup(Counter 0|Counter 1|Both),edit,edit
      mask Display: disp('PXI-6070E\nNational Instr.\nPulse Gen.');port_label('input', 1, '0');
  PXI-6070E 1 : S-Function  InitFcn=mctrnipciecap(1);  FunctionName=pwmnipcie  Parameters=channel, trigmd, polarity, tsamp, slot, boardType  mask(pwmnipxi6070e){channel=0, trigmd=Level Triggered, polarity=Active low, tsamp=0.01, slot=-1}
      mask prompts: channel "Counter:"; trigmd "Trigger mode:"; tsamp "Sample time:"; slot "PCI slot (-1: autosearch):"
      mask help:
      | PXI-6070E
      | National Instruments
      | Pulsewidth/Period measurement
      mask init:
      | boardType = 6;
      | 
      | channel  = channel  - 1;
      | trigmd   = trigmd   - 1;
      | polarity = polarity - 1;
      | mctrnipciecap(2, boardType, slot, channel);
      mask Help: helpview(fullfile(docroot, 'mapfiles', 'xpc.map'),'NationalInstruments_PXI-6070E_CTRMEAS');
      mask StyleString: popup(0|1),popup(Level Triggered|Edge Triggered),popup(Active low|Active high),edit,edit
      mask CallbackString: |mnipwmmaskenable(gcb)|||
      mask Display: disp('PXI-6070E\nNational Instr.\nPulsewidth/Period Meas.');port_label('output', 1, '0');
  "PXI-6071E " : S-Function  FunctionName=ctrnipcie  Parameters=channel, sampletime, slot, boardType  mask(ctrnipxi6071e){channel=Counter 0, sampletime=-1, slot=-1}
      mask prompts: channel "Counter:"; sampletime "Sample time:"; slot "PCI slot (-1: autosearch):"
      mask help:
      | PXI-6071E
      | National Instruments
      | Pulse Generation
      mask init:
      | boardType = 12;
      | mctrnipcie(2, boardType, slot, channel);
      mask Help: helpview(fullfile(docroot, 'mapfiles', 'xpc.map'),'NationalInstruments_PXI-6071E_CTR');
      mask StyleString: popup(Counter 0|Counter 1|Both),edit,edit
      mask Display: disp('PXI-6071E\nNational Instr.\nPulse Gen.');port_label('input', 1, '0');
  PXI-6071E 1 : S-Function  InitFcn=mctrnipciecap(1);  FunctionName=pwmnipcie  Parameters=channel, trigmd, polarity, tsamp, slot, boardType  mask(pwmnipxi6071e){channel=0, trigmd=Level Triggered, polarity=Active low, tsamp=0.01, slot=-1}
      mask prompts: channel "Counter:"; trigmd "Trigger mode:"; tsamp "Sample time:"; slot "PCI slot (-1: autosearch):"
      mask help:
      | PXI-6071E
      | National Instruments
      | Pulsewidth/Period measurement
      mask init:
      | boardType = 12;
      | 
      | channel  = channel  - 1;
      | trigmd   = trigmd   - 1;
      | polarity = polarity - 1;
      | mctrnipciecap(2, boardType, slot, channel);
      mask Help: helpview(fullfile(docroot, 'mapfiles', 'xpc.map'),'NationalInstruments_PXI-6071E_CTRMEAS');
      mask StyleString: popup(0|1),popup(Level Triggered|Edge Triggered),popup(Active low|Active high),edit,edit
      mask CallbackString:
      | |mv = get_param(gcb, 'MaskValues');
      | me = get_param(gcb, 'MaskEnables');
      | if strncmp(mv{2}, 'Level', 4)
      | 	me{3} = 'on';
      | else
      | 	me{3} = 'off';
      | end
      | set_param(gcb, 'MaskEnables', me);|||
      mask Display: disp('PXI-6071E\nNational Instr.\nPulsewidth/Period Meas.');port_label('output', 1, '0');
  PXI6602 1 : S-Function  InitFcn=mnipci660x(1);  FunctionName=pwmnipci660x  Parameters=channel, trigmd, polarity, tsamp, slot, boardType  mask(pwmnipxi6602){channel=1, trigmd=Level Triggered, polarity=Active Low, tsamp=0.001, slot=-1}
      mask prompts: trigmd "Trigger mode:"; tsamp "Sample time:"; slot "PCI slot (-1: autosearch):"
      mask help:
      | PXI-6602
      | National Instruments
      | Pulsewidth/Period Measurement
      mask init:
      | boardType = 2;
      | 
      | channel  = channel  - 1;
      | trigmd   = trigmd   - 1;
      | polarity = polarity - 1;
      | mnipci660x( 2, channel, slot, boardType )
      mask Help: helpview(fullfile(docroot, 'mapfiles', 'xpc.map'), 'NationalInstruments_PCI-6602_CTRMEAS')
      mask StyleString: popup(1|2|3|4|5|6|7|8),popup(Level Triggered|Edge Triggered),popup(Active Low|Active High),edit,edit
      mask CallbackString: |mnipwmmaskenable(gcb);|||
      mask Display:
      | disp('PXI-6602\nNational Instr.\nPulsewidth/Period Meas.');
      | port_label('output', 1, 'C');
